simulink model "px4demo_attitude_system_multi_task"  (R2014b)
settings: Solver=FixedStepDiscrete  SolverMode=SingleTasking  StartTime=0.0  StopTime=inf  RelTol=1e-3
PostLoadFcn:
  | kFactor = 1.2;
  | 
  | KpRollAttitude = 0.630138625117681 / kFactor;
  | KiRollAttitude = 0.0552303199591522 / kFactor;
  | 
  | KpPitchAttitude = 0.630138625117681 / kFactor;
  | KiPitchAttitude = 0.0552303199591522 / kFactor;
  | 
  | KpRollRate = 1.31533836563383 / kFactor;
  | KiRollRate = 0.460338699849681 / kFactor;
  | 
  | KpPitchRate = 1.31533836563383 / kFactor;
  | KiPitchRate = 0.460338699849681 / kFactor;
  | 
  | KpYawRate = 1.31533836563383 / kFactor;
  | KiYawRate = 0.460338699849681 / kFactor;
undefined symbols (not defined in the file): PX4_TUNE_ENUM, RGBLED_COLOR_ENUM, RGBLED_MODE_ENUM
libraries: simulink x6, pixhawk_sllib x6
settings Model: SimulationMode=external  ExtModeTrigDuration=800  ExtModeArchiveFileName=EXT_mode_log  ExtModeArchiveDirName=C:\Pixhawk_Branch_Experiment\Ext_mode_bkgnd\Data_Logging  ExtModeAddSuffixToVar=on  ExtModeWriteAllDataToWs=on  ExtModeLogAll=off  Creator=Adam  LastModifiedBy=darenlee
settings SolverCC: AutoInsertRateTranBlk=on
settings OptimizationCC: InlineParams=on  OptimizeModelRefInitCode=on  LifeSpan=1  MaxStackSize=64
settings HardwareCC: ProdLargestAtomicInteger=Long  ProdLargestAtomicFloat=Double  ProdEndianess=LittleEndian  ProdHWDeviceType=ARM Compatible->ARM Cortex
settings RTWCC: SystemTargetFile=ert.tlc  TemplateMakefile=ert_default_tmf  Description=Embedded Coder  GenerateReport=on  ProcessScript=ert_make_rtw_hook  Toolchain=Pixhawk Toolchain  IncludeHyperlinkInReport=on  LaunchReport=on  GenerateTraceReport=on  GenerateTraceReportSl=on  GenerateTraceReportSf=on  GenerateTraceReportEml=on  GenerateCodeMetricsReport=on
settings CodeAppCC: IgnoreCustomStorageClasses=off
settings ERTTargetCC: CodeReplacementLibrary=GCC ARM Cortex-A9  ExtMode=on  ExtModeTransport=1  ExtModeMexFile=ext_serial_win32_comm  ExtModeMexArgs=1 8 57600 10  ERTCustomFileTemplate=PX4_codertarget_file_process.tlc

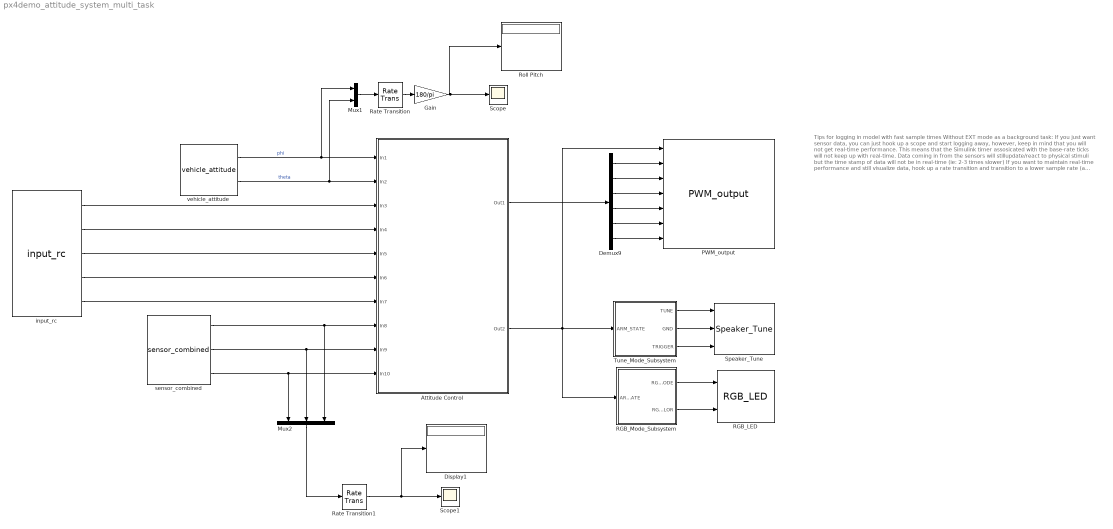
== system px4demo_attitude_system_multi_task ==
  note: Tips for logging in model with fast sample times
      |
      | Without EXT mode as a background task:
      | If you just want sensor data, you can just hook up a scope and start logging away, however, keep in mind that you will not get real-time performance. This means that the Simulink timer assosicated with the base-rate ticks will not keep up with real-time. Data coming in from the sensors will stillupdate/react to physical stimuli but the time stamp of data will not be in real-time (ie: 2-3 times slower)
      |
      | If you want to maintain real-time performance and still visualize data, hook up a rate transition and transition to a lower sample rate (a factor of 10 lower) and set the duration size to a value that will not cause the clock to slow down that much
      |
      | Recall that duration is the number of base-rate 'ticks' of data to give back. Sometimes if you set the duration too low data fails to come in for a specified sample rate. For instance, if we chose a duration value of 1:
      | 1 * 0.004 = 0.004 seconds worth of data
      | What will the lower sample (0.04s) scope show?
      | int( 0.004/0.04 ) = 0.. if we check the scope we see no data
      |
      | However, if we chose a duration value of 20
      | 400*0.004 = 1.6 seconds worth of data from base-rate
      | 1.60 / 0.04 = 40 points of data on the lower sample time scopes
      |
      | In other words, ensure the number of duration ticks gives you enough data
      | points to view on the lower sample rates, otherwise you wont see any data at all. Consult the documentation for more detail
      |
      | Using EXT mode with background task enabled
      |
      | This model has already been configured to use a background task and already uses a lot of the tips described in the above steps. With background tasking, the base-rate task is not encumbered by having to run external mode tasks at the same time, instead, EXT mode is now running in the background on another task being paced at 10 Hz. This can greatly help with real-time performance. Sometimes you may want to use the default behavior if you only have a single sample-time running at a slow rate - if you want data to come in faster or as fast as the model's sample-time then you'll want to use default behavior. On the other hand, if your model is running with multiple rates at varying speeds, you will want to pick the back-ground task option
  Attitude Control : Subsystem
  Demux9 : Demux  Outputs=6
  Display1 : Display
  Gain : Gain  Gain=180/pi
  Mux1 : Mux  Inputs=2
  Mux2 : Mux  Inputs=3
  PWM_output : pixhawk_sllib/PWM_output  show_pwm1=on  show_pwm2=on  show_pwm3=on  show_pwm4=on  show_pwm5=on  show_pwm6=on  show_pwm7=off  show_pwm8=off
  RGB_LED : pixhawk_sllib/RGB_LED
  RGB_Mode_Subsystem : Subsystem
  Rate Transition : RateTransition  OutPortSampleTime=0.04
  Rate Transition1 : RateTransition  OutPortSampleTime=0.04
  Roll Pitch : Display
  Scope : Scope
      settings: TimeRange=2  YMin=-1  YMax=1
  Scope1 : Scope
      settings: TimeRange=1.5  YMin=-1  YMax=1
  Speaker_Tune : pixhawk_sllib/Speaker_Tune
  Tune_Mode_Subsystem : Subsystem
  input_rc : pixhawk_sllib/input_rc  sampletime=1/250  channel1=on  channel2=on  channel3=on  channel4=on  channel5=on  channel6=off  channel7=off  channel8=off  ch_count=off  rssi=off  rc_failsafe=off  rc_lost=off  rc_inputsource=off
  sensor_combined : pixhawk_sllib/sensor_combined  sampletime=1/250  show_mag=off  show_acc=off  show_gyro=on  show_baro=off  show_ts=off
  vehicle_attitude : pixhawk_sllib/vehicle_attitude  sampletime=1/250  show_r=on  show_p=on  show_y=off  show_q=off
  wires:
  Demux9/6 -> PWM_output/7
  Demux9/5 -> PWM_output/6
  Demux9/4 -> PWM_output/5
  Demux9/2 -> PWM_output/3
  Demux9/3 -> PWM_output/4
  RGB_Mode_Subsystem/1(RGB_MODE) -> RGB_LED/1
  RGB_Mode_Subsystem/2(RGB_COLOR) -> RGB_LED/2
  Tune_Mode_Subsystem/1(TUNE) -> Speaker_Tune/1
  Tune_Mode_Subsystem/2(GND) -> Speaker_Tune/2
  Tune_Mode_Subsystem/3(TRIGGER) -> Speaker_Tune/3
  Attitude Control/2(Out2) -> PWM_output/1, Tune_Mode_Subsystem/1(ARM_STATE), RGB_Mode_Subsystem/1(ARM_STATE)
  vehicle_attitude/1 -> Mux1/1, Attitude Control/1(In1)  "phi"
  vehicle_attitude/2 -> Attitude Control/2(In2), Mux1/2  "theta"
  input_rc/1 -> Attitude Control/3(In3)
  input_rc/2 -> Attitude Control/4(In4)
  input_rc/3 -> Attitude Control/5(In5)
  input_rc/4 -> Attitude Control/6(In6)
  sensor_combined/1 -> Mux2/3, Attitude Control/8(In8)
  sensor_combined/2 -> Mux2/2, Attitude Control/9(In9)
  sensor_combined/3 -> Mux2/1, Attitude Control/10(In10)
  Attitude Control/1(Out1) -> Demux9/1
  Demux9/1 -> PWM_output/2
  input_rc/5 -> Attitude Control/7(In7)
  Mux1/1 -> Rate Transition/1
  Rate Transition/1 -> Gain/1
  Rate Transition1/1 -> Scope1/1, Display1/1
  Mux2/1 -> Rate Transition1/1
  Gain/1 -> Roll Pitch/1, Scope/1

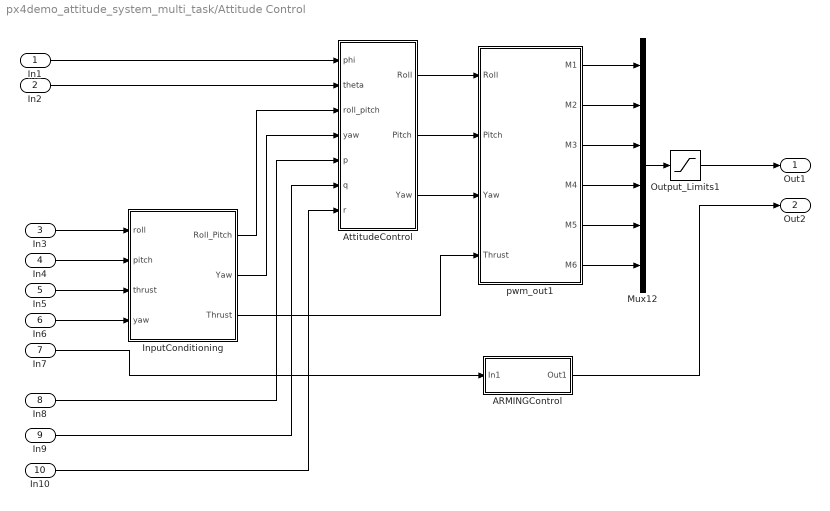
== system px4demo_attitude_system_multi_task/Attitude Control ==
  In1 : Inport
  In2 : Inport  Port=2
  In3 : Inport  Port=3
  In4 : Inport  Port=4
  In5 : Inport  Port=5
  In6 : Inport  Port=6
  In7 : Inport  Port=7
  In8 : Inport  Port=8
  In9 : Inport  Port=9
  In10 : Inport  Port=10
  ARMINGControl : Subsystem
  AttitudeControl : Subsystem
  InputConditioning : Subsystem
  Mux12 : Mux  Inputs=6
  Output_Limits1 : Saturate  UpperLimit=2000  LowerLimit=1000
  pwm_out1 : MATLAB Function  TreatAsAtomicUnit=on  SystemSampleTime=0.004
  Out1 : Outport
  Out2 : Outport  Port=2
  wires:
  ARMINGControl/1(Out1) -> Out2/1
  In6/1 -> InputConditioning/4(yaw)
  pwm_out1/4(M4) -> Mux12/4
  pwm_out1/3(M3) -> Mux12/3
  pwm_out1/2(M2) -> Mux12/2
  pwm_out1/1(M1) -> Mux12/1
  pwm_out1/5(M5) -> Mux12/5
  In7/1 -> ARMINGControl/1(In1)
  AttitudeControl/3(Yaw) -> pwm_out1/3(Yaw)
  AttitudeControl/2(Pitch) -> pwm_out1/2(Pitch)
  AttitudeControl/1(Roll) -> pwm_out1/1(Roll)
  In10/1 -> AttitudeControl/7(r)
  In9/1 -> AttitudeControl/6(q)
  In8/1 -> AttitudeControl/5(p)
  InputConditioning/2(Yaw) -> AttitudeControl/4(yaw)
  InputConditioning/1(Roll_Pitch) -> AttitudeControl/3(roll_pitch)
  In2/1 -> AttitudeControl/2(theta)
  In1/1 -> AttitudeControl/1(phi)
  InputConditioning/3(Thrust) -> pwm_out1/4(Thrust)
  Output_Limits1/1 -> Out1/1
  Mux12/1 -> Output_Limits1/1
  In4/1 -> InputConditioning/2(pitch)
  In3/1 -> InputConditioning/1(roll)
  pwm_out1/6(M6) -> Mux12/6
  In5/1 -> InputConditioning/3(thrust)

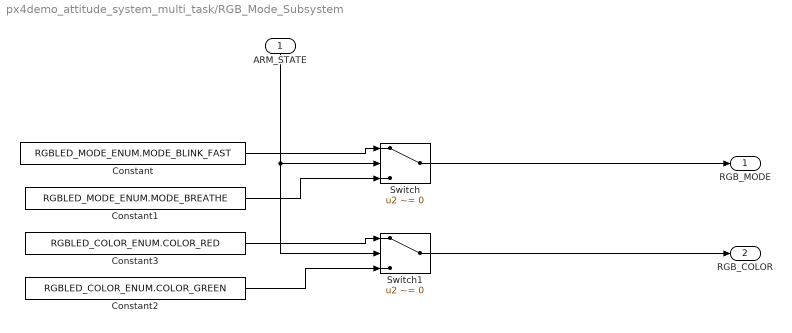
== system px4demo_attitude_system_multi_task/RGB_Mode_Subsystem ==
  ARM_STATE : Inport
  Constant : Constant  Value=RGBLED_MODE_ENUM.MODE_BLINK_FAST  OutDataTypeStr=Enum: RGBLED_MODE_ENUM
  Constant1 : Constant  Value=RGBLED_MODE_ENUM.MODE_BREATHE  OutDataTypeStr=Enum: RGBLED_MODE_ENUM
  Constant2 : Constant  Value=RGBLED_COLOR_ENUM.COLOR_GREEN  OutDataTypeStr=Enum: RGBLED_COLOR_ENUM
  Constant3 : Constant  Value=RGBLED_COLOR_ENUM.COLOR_RED  OutDataTypeStr=Enum: RGBLED_COLOR_ENUM
  Switch : Switch  Criteria=u2 ~= 0  Threshold=1500  SampleTime=1/2
  Switch1 : Switch  Criteria=u2 ~= 0  Threshold=1500  SampleTime=1/2
  RGB_MODE : Outport
  RGB_COLOR : Outport  Port=2
  wires:
  ARM_STATE/1 -> Switch1/2, Switch/2
  Constant/1 -> Switch/1
  Constant1/1 -> Switch/3
  Switch/1 -> RGB_MODE/1
  Constant3/1 -> Switch1/1
  Constant2/1 -> Switch1/3
  Switch1/1 -> RGB_COLOR/1

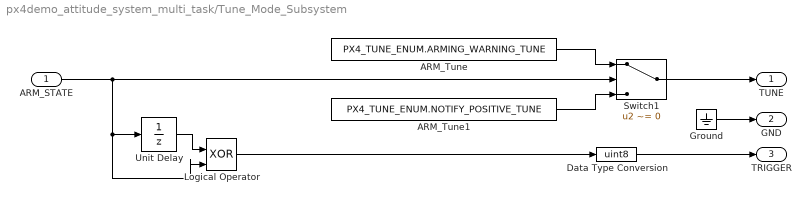
== system px4demo_attitude_system_multi_task/Tune_Mode_Subsystem ==
  ARM_STATE : Inport
  ARM_Tune : Constant  Value=PX4_TUNE_ENUM.ARMING_WARNING_TUNE  OutDataTypeStr=Enum: PX4_TUNE_ENUM
  ARM_Tune1 : Constant  Value=PX4_TUNE_ENUM.NOTIFY_POSITIVE_TUNE  OutDataTypeStr=Enum: PX4_TUNE_ENUM
  Data Type Conversion : DataTypeConversion  OutDataTypeStr=uint8
  Ground : Ground
  Logical Operator : Logic  Operator=XOR  IconShape=distinctive  AllPortsSameDT=off  OutDataTypeStr=boolean
  Switch1 : Switch  Criteria=u2 ~= 0  Threshold=1500
  Unit Delay : UnitDelay  SampleTime=-1
  TUNE : Outport
  GND : Outport  Port=2
  TRIGGER : Outport  Port=3
  wires:
  Ground/1 -> GND/1
  Data Type Conversion/1 -> TRIGGER/1
  Switch1/1 -> TUNE/1
  ARM_Tune/1 -> Switch1/1
  ARM_Tune1/1 -> Switch1/3
  ARM_STATE/1 -> Logical Operator/2, Unit Delay/1, Switch1/2
  Unit Delay/1 -> Logical Operator/1
  Logical Operator/1 -> Data Type Conversion/1

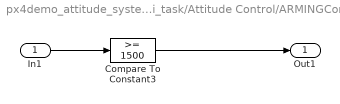
== system px4demo_attitude_system_multi_task/Attitude Control/ARMINGControl ==
  In1 : Inport
  Compare To Constant3 : simulink/Logic and Bit Operations/Compare To Constant  relop=>=  const=1500  OutDataTypeStr=boolean
  Out1 : Outport
  wires:
  Compare To Constant3/1 -> Out1/1
  In1/1 -> Compare To Constant3/1

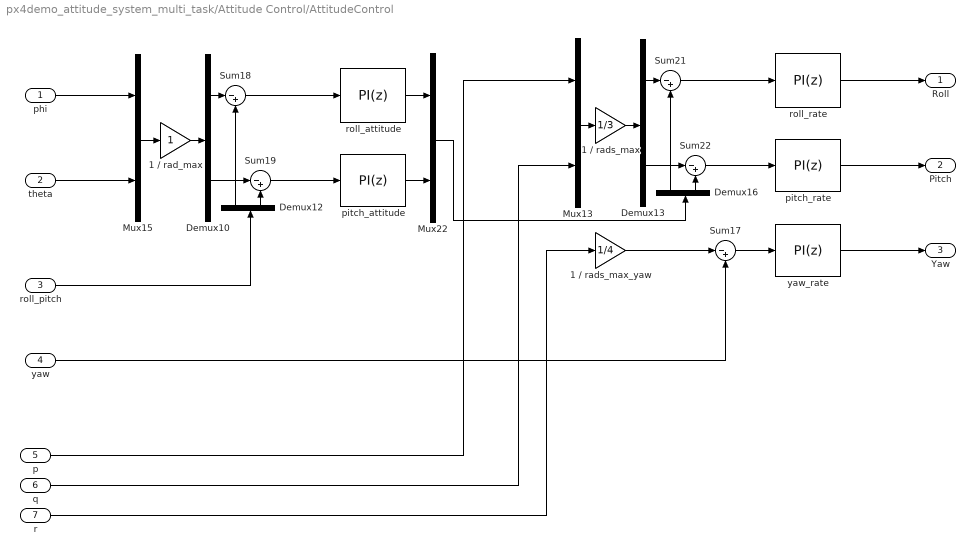
== system px4demo_attitude_system_multi_task/Attitude Control/AttitudeControl ==
  phi : Inport
  theta : Inport  Port=2
  roll_pitch : Inport  Port=3
  yaw : Inport  Port=4
  p : Inport  Port=5
  q : Inport  Port=6
  r : Inport  Port=7
  1 / rad_max : Gain
  1 / rads_max : Gain  Gain=1/3
  1 / rads_max_yaw : Gain  Gain=1/4
  Demux{10,12..13,16} (4 alike) : Demux  Outputs=2
  Mux13 : Mux  Inputs=2
  Mux15 : Mux  Inputs=2
  Mux22 : Mux  Inputs=2
  Sum{17..19,21..22} (5 alike) : Sum  Inputs=|-+
  pitch_attitude : simulink/Continuous/PID Controller  Controller=PI  TimeDomain=Discrete-time  SampleTime=-1  IntegratorMethod=Forward Euler  FilterMethod=Forward Euler  Form=Parallel  P=KpPitchAttitude  I=KiPitchAttitude  D=0.01  N=100  InitialConditionSource=internal  InitialConditionForIntegrator=0  InitialConditionForFilter=0  ExternalReset=none  LimitOutput=on  UpperSaturationLimit=1  LowerSaturationLimit=-1  LinearizeAsGain=on  AntiWindupMode=back-calculation  Kb=1  TrackingMode=off  Kt=1  PParamMin=[]  PParamMax=[]  IParamMin=[]  IParamMax=[]  DParamMin=[]  DParamMax=[]  NParamMin=[]  NParamMax=[]  KbParamMin=[]  KbParamMax=[]  KtParamMin=[]  KtParamMax=[]  POutMin=[]  POutMax=[]  IOutMin=[]  IOutMax=[]  DOutMin=[]  DOutMax=[]  NOutMin=[]  NOutMax=[]  KbOutMin=[]  KbOutMax=[]  KtOutMin=[]  KtOutMax=[]  IntegratorOutMin=[]  IntegratorOutMax=[]  FilterOutMin=[]  FilterOutMax=[]  SumOutMin=[]  SumOutMax=[]  SumI1OutMin=[]  SumI1OutMax=[]  SumI2OutMin=[]  SumI2OutMax=[]  SumI3OutMin=[]  SumI3OutMax=[]  SumDOutMin=[]  SumDOutMax=[]  SaturationOutMin=[]  SaturationOutMax=[]  IntegratorContinuousStateAttributes=''  IntegratorStateMustResolveToSignalObject=off  IntegratorRTWStateStorageClass=Auto  FilterContinuousStateAttributes=''  FilterStateMustResolveToSignalObject=off  FilterRTWStateStorageClass=Auto  DifferentiatorICPrevScaledInput=0  DifferentiatorOutMin=[]  DifferentiatorOutMax=[]  UseFilter=on
  pitch_rate : simulink/Continuous/PID Controller  Controller=PI  TimeDomain=Discrete-time  SampleTime=-1  IntegratorMethod=Forward Euler  FilterMethod=Forward Euler  Form=Parallel  P=KpPitchRate  I=KiPitchRate  D=0.0024  N=100  InitialConditionSource=internal  InitialConditionForIntegrator=0  InitialConditionForFilter=0  ExternalReset=none  LimitOutput=on  UpperSaturationLimit=1  LowerSaturationLimit=-1  LinearizeAsGain=on  AntiWindupMode=back-calculation  Kb=1  TrackingMode=off  Kt=1  PParamMin=[]  PParamMax=[]  IParamMin=[]  IParamMax=[]  DParamMin=[]  DParamMax=[]  NParamMin=[]  NParamMax=[]  KbParamMin=[]  KbParamMax=[]  KtParamMin=[]  KtParamMax=[]  POutMin=[]  POutMax=[]  IOutMin=[]  IOutMax=[]  DOutMin=[]  DOutMax=[]  NOutMin=[]  NOutMax=[]  KbOutMin=[]  KbOutMax=[]  KtOutMin=[]  KtOutMax=[]  IntegratorOutMin=[]  IntegratorOutMax=[]  FilterOutMin=[]  FilterOutMax=[]  SumOutMin=[]  SumOutMax=[]  SumI1OutMin=[]  SumI1OutMax=[]  SumI2OutMin=[]  SumI2OutMax=[]  SumI3OutMin=[]  SumI3OutMax=[]  SumDOutMin=[]  SumDOutMax=[]  SaturationOutMin=[]  SaturationOutMax=[]  IntegratorContinuousStateAttributes=''  IntegratorStateMustResolveToSignalObject=off  IntegratorRTWStateStorageClass=Auto  FilterContinuousStateAttributes=''  FilterStateMustResolveToSignalObject=off  FilterRTWStateStorageClass=Auto  DifferentiatorICPrevScaledInput=0  DifferentiatorOutMin=[]  DifferentiatorOutMax=[]  UseFilter=on
  roll_attitude : simulink/Continuous/PID Controller  Controller=PI  TimeDomain=Discrete-time  SampleTime=-1  IntegratorMethod=Forward Euler  FilterMethod=Forward Euler  Form=Parallel  P=KpRollAttitude  I=KiRollAttitude  D=0.01  N=100  InitialConditionSource=internal  InitialConditionForIntegrator=0  InitialConditionForFilter=0  ExternalReset=none  LimitOutput=on  UpperSaturationLimit=1  LowerSaturationLimit=-1  LinearizeAsGain=on  AntiWindupMode=back-calculation  Kb=1  TrackingMode=off  Kt=1  PParamMin=[]  PParamMax=[]  IParamMin=[]  IParamMax=[]  DParamMin=[]  DParamMax=[]  NParamMin=[]  NParamMax=[]  KbParamMin=[]  KbParamMax=[]  KtParamMin=[]  KtParamMax=[]  POutMin=[]  POutMax=[]  IOutMin=[]  IOutMax=[]  DOutMin=[]  DOutMax=[]  NOutMin=[]  NOutMax=[]  KbOutMin=[]  KbOutMax=[]  KtOutMin=[]  KtOutMax=[]  IntegratorOutMin=[]  IntegratorOutMax=[]  FilterOutMin=[]  FilterOutMax=[]  SumOutMin=[]  SumOutMax=[]  SumI1OutMin=[]  SumI1OutMax=[]  SumI2OutMin=[]  SumI2OutMax=[]  SumI3OutMin=[]  SumI3OutMax=[]  SumDOutMin=[]  SumDOutMax=[]  SaturationOutMin=[]  SaturationOutMax=[]  IntegratorContinuousStateAttributes=''  IntegratorStateMustResolveToSignalObject=off  IntegratorRTWStateStorageClass=Auto  FilterContinuousStateAttributes=''  FilterStateMustResolveToSignalObject=off  FilterRTWStateStorageClass=Auto  DifferentiatorICPrevScaledInput=0  DifferentiatorOutMin=[]  DifferentiatorOutMax=[]  UseFilter=on
  roll_rate : simulink/Continuous/PID Controller  Controller=PI  TimeDomain=Discrete-time  SampleTime=-1  IntegratorMethod=Forward Euler  FilterMethod=Forward Euler  Form=Parallel  P=KpRollRate  I=KiRollRate  D=0.0024  N=100  InitialConditionSource=internal  InitialConditionForIntegrator=0  InitialConditionForFilter=0  ExternalReset=none  LimitOutput=on  UpperSaturationLimit=1  LowerSaturationLimit=-1  LinearizeAsGain=on  AntiWindupMode=back-calculation  Kb=1  TrackingMode=off  Kt=1  PParamMin=[]  PParamMax=[]  IParamMin=[]  IParamMax=[]  DParamMin=[]  DParamMax=[]  NParamMin=[]  NParamMax=[]  KbParamMin=[]  KbParamMax=[]  KtParamMin=[]  KtParamMax=[]  POutMin=[]  POutMax=[]  IOutMin=[]  IOutMax=[]  DOutMin=[]  DOutMax=[]  NOutMin=[]  NOutMax=[]  KbOutMin=[]  KbOutMax=[]  KtOutMin=[]  KtOutMax=[]  IntegratorOutMin=[]  IntegratorOutMax=[]  FilterOutMin=[]  FilterOutMax=[]  SumOutMin=[]  SumOutMax=[]  SumI1OutMin=[]  SumI1OutMax=[]  SumI2OutMin=[]  SumI2OutMax=[]  SumI3OutMin=[]  SumI3OutMax=[]  SumDOutMin=[]  SumDOutMax=[]  SaturationOutMin=[]  SaturationOutMax=[]  IntegratorContinuousStateAttributes=''  IntegratorStateMustResolveToSignalObject=off  IntegratorRTWStateStorageClass=Auto  FilterContinuousStateAttributes=''  FilterStateMustResolveToSignalObject=off  FilterRTWStateStorageClass=Auto  DifferentiatorICPrevScaledInput=0  DifferentiatorOutMin=[]  DifferentiatorOutMax=[]  UseFilter=on
  yaw_rate : simulink/Continuous/PID Controller  Controller=PI  TimeDomain=Discrete-time  SampleTime=-1  IntegratorMethod=Forward Euler  FilterMethod=Forward Euler  Form=Parallel  P=KpYawRate  I=KiYawRate  D=0  N=100  InitialConditionSource=internal  InitialConditionForIntegrator=0  InitialConditionForFilter=0  ExternalReset=none  LimitOutput=on  UpperSaturationLimit=1  LowerSaturationLimit=-1  LinearizeAsGain=on  AntiWindupMode=back-calculation  Kb=1  TrackingMode=off  Kt=1  PParamMin=[]  PParamMax=[]  IParamMin=[]  IParamMax=[]  DParamMin=[]  DParamMax=[]  NParamMin=[]  NParamMax=[]  KbParamMin=[]  KbParamMax=[]  KtParamMin=[]  KtParamMax=[]  POutMin=[]  POutMax=[]  IOutMin=[]  IOutMax=[]  DOutMin=[]  DOutMax=[]  NOutMin=[]  NOutMax=[]  KbOutMin=[]  KbOutMax=[]  KtOutMin=[]  KtOutMax=[]  IntegratorOutMin=[]  IntegratorOutMax=[]  FilterOutMin=[]  FilterOutMax=[]  SumOutMin=[]  SumOutMax=[]  SumI1OutMin=[]  SumI1OutMax=[]  SumI2OutMin=[]  SumI2OutMax=[]  SumI3OutMin=[]  SumI3OutMax=[]  SumDOutMin=[]  SumDOutMax=[]  SaturationOutMin=[]  SaturationOutMax=[]  IntegratorContinuousStateAttributes=''  IntegratorStateMustResolveToSignalObject=off  IntegratorRTWStateStorageClass=Auto  FilterContinuousStateAttributes=''  FilterStateMustResolveToSignalObject=off  FilterRTWStateStorageClass=Auto  DifferentiatorICPrevScaledInput=0  DifferentiatorOutMin=[]  DifferentiatorOutMax=[]  UseFilter=on
  Roll : Outport
  Pitch : Outport  Port=2
  Yaw : Outport  Port=3
  wires:
  r/1 -> 1 / rads_max_yaw/1
  q/1 -> Mux13/2
  Mux22/1 -> Demux16/1
  yaw_rate/1 -> Yaw/1
  phi/1 -> Mux15/1
  Mux15/1 -> 1 / rad_max/1
  theta/1 -> Mux15/2
  1 / rads_max_yaw/1 -> Sum17/1
  roll_rate/1 -> Roll/1
  Sum19/1 -> pitch_attitude/1
  pitch_attitude/1 -> Mux22/2
  roll_attitude/1 -> Mux22/1
  Demux16/1 -> Sum21/2
  yaw/1 -> Sum17/2
  roll_pitch/1 -> Demux12/1
  Demux16/2 -> Sum22/2
  Demux12/1 -> Sum18/2
  Demux12/2 -> Sum19/2
  p/1 -> Mux13/1
  Demux10/1 -> Sum18/1
  Demux10/2 -> Sum19/1
  1 / rad_max/1 -> Demux10/1
  Sum18/1 -> roll_attitude/1
  pitch_rate/1 -> Pitch/1
  Mux13/1 -> 1 / rads_max/1
  Sum22/1 -> pitch_rate/1
  Sum17/1 -> yaw_rate/1
  Demux13/1 -> Sum21/1
  Demux13/2 -> Sum22/1
  1 / rads_max/1 -> Demux13/1
  Sum21/1 -> roll_rate/1

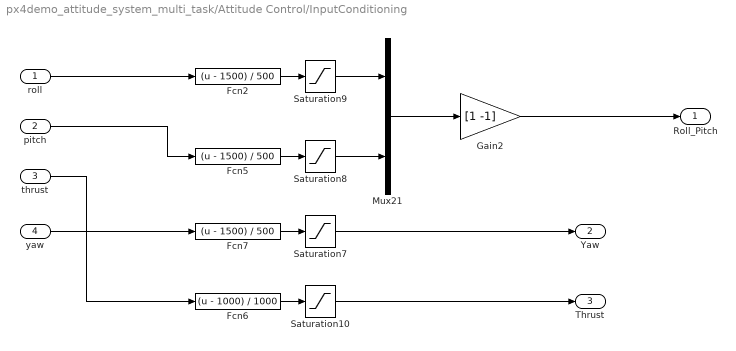
== system px4demo_attitude_system_multi_task/Attitude Control/InputConditioning ==
  roll : Inport
  pitch : Inport  Port=2
  thrust : Inport  Port=3
  yaw : Inport  Port=4
  Fcn2 : Fcn  Expr=(u - 1500) / 500
  Fcn5 : Fcn  Expr=(u - 1500) / 500
  Fcn6 : Fcn  Expr=(u - 1000) / 1000
  Fcn7 : Fcn  Expr=(u - 1500) / 500
  Gain2 : Gain  Gain=[1 -1]
  Mux21 : Mux  Inputs=2
  Saturation10 : Saturate  UpperLimit=1  LowerLimit=0
  Saturation7 : Saturate  UpperLimit=1  LowerLimit=-1
  Saturation8 : Saturate  UpperLimit=1  LowerLimit=-1
  Saturation9 : Saturate  UpperLimit=1  LowerLimit=-1
  Roll_Pitch : Outport
  Yaw : Outport  Port=2
  Thrust : Outport  Port=3
  wires:
  Saturation10/1 -> Thrust/1
  Saturation7/1 -> Yaw/1
  Gain2/1 -> Roll_Pitch/1
  Mux21/1 -> Gain2/1
  Saturation8/1 -> Mux21/2
  Fcn6/1 -> Saturation10/1
  thrust/1 -> Fcn6/1
  Fcn2/1 -> Saturation9/1
  Fcn5/1 -> Saturation8/1
  Saturation9/1 -> Mux21/1
  Fcn7/1 -> Saturation7/1
  yaw/1 -> Fcn7/1
  pitch/1 -> Fcn5/1
  roll/1 -> Fcn2/1

== matlab function px4demo_attitude_system_multi_task/Attitude Control/pwm_out1 ==
  data: Roll input; M1 output; Pitch input; Yaw input; Thrust input; M2 output; M3 output; M4 output; M5 output; M6 output
function [M1, M2, M3, M4, M5, M6] = motor_mixer(Roll, Pitch, Yaw, Thrust)

idle_PWM = 1000;

% Quad X
% M1 = ((Roll + Pitch - Yaw) / 2 * Thrust + Thrust) * 1000 + idle_PWM;
% M2 = ((-Roll + Pitch + Yaw) / 2 * Thrust + Thrust) * 1000 + idle_PWM;
% M3 = ((-Roll - Pitch - Yaw) / 2 * Thrust + Thrust) * 1000 + idle_PWM;
% M4 = ((Roll - Pitch + Yaw) / 2 * Thrust + Thrust) * 1000 + idle_PWM;
% M5 = 1000;
% M6 = 1000;
% M7 = 1000;
% M8 = 1000;

% Quad +
% M1 = ((Pitch - Yaw) * Thrust / 2 + Thrust) * 1000 + idle_PWM;
% M2 = ((-Roll + Yaw) * Thrust / 2 + Thrust) * 1000 + idle_PWM;
% M3 = ((-Pitch - Yaw) * Thrust / 2 + Thrust) * 1000 + idle_PWM;
% M4 = ((Roll + Yaw) * Thrust / 2 + Thrust) * 1000 + idle_PWM;
% M5 = 1000;
% M6 = 1000;
% M7 = 1000;
% M8 = 1000;

% Hex X
% M1 = ((Pitch + Roll / 2 - Yaw) * Thrust / 2 + Thrust) * 1000 + idle_PWM;
% M2 = ((Pitch - Roll / 2 + Yaw) * Thrust / 2 + Thrust) * 1000 + idle_PWM;
% M3 = ((-Roll - Yaw) * Thrust / 2 + Thrust) * 1000 + idle_PWM;
% M4 = ((-Pitch - Roll / 2 + Yaw) * Thrust / 2 + Thrust) * 1000 + idle_PWM;
% M5 = ((-Pitch + Roll / 2 - Yaw) * Thrust / 2 + Thrust) * 1000 + idle_PWM;
% M6 = ((Roll + Yaw) * Thrust / 2 + Thrust) * 1000 + idle_PWM;
% M7 = 1000;
% M8 = 1000;

% My Hex X (From Adam)
% 1M3 = ((-Roll - Yaw) * Thrust / 2 + Thrust) * 1000 + idle_PWM;
% 2M6 = ((Roll + Yaw) * Thrust / 2 + Thrust) * 1000 + idle_PWM;
% 3M1 = ((Pitch + Roll / 2 - Yaw) * Thrust / 2 + Thrust) * 1000 + idle_PWM;
% 4M4 = ((-Pitch - Roll / 2 + Yaw) * Thrust / 2 + Thrust) * 1000 + idle_PWM;
% 5M2 = ((Pitch - Roll / 2 + Yaw) * Thrust / 2 + Thrust) * 1000 + idle_PWM;
% 6M5 = ((-Pitch + Roll / 2 - Yaw) * Thrust / 2 + Thrust) * 1000 + idle_PWM;
M1 = ((-Roll - Yaw) * Thrust / 3 + Thrust) * 1000 + idle_PWM;
M2 = ((Roll + Yaw) * Thrust / 3 + Thrust) * 1000 + idle_PWM;
M3 = ((Pitch + Roll / 2 - Yaw) * Thrust / 3 + Thrust) * 1000 + idle_PWM;
M4 = ((-Pitch - Roll / 2 + Yaw) * Thrust / 3 + Thrust) * 1000 + idle_PWM;
M5 = ((Pitch - Roll / 2 + Yaw) * Thrust / 3 + Thrust) * 1000 + idle_PWM;
M6 = ((-Pitch + Roll / 2 - Yaw) * Thrust / 3 + Thrust) * 1000 + idle_PWM;

% My Hex X (Version 2)
% Roll/Yaw
% M1 = ((-Roll - Yaw) * Thrust / 2 + Thrust) * 1000 + idle_PWM;
% M2 = ((Roll + Yaw) * Thrust / 2 + Thrust) * 1000 + idle_PWM;
% % + Pitch/Roll
% M6 = ((Pitch + Roll / 2 - Yaw) * Thrust / 2 + Thrust) * 1000 + idle_PWM;
% M4 = ((Pitch - Roll / 2 + Yaw) * Thrust / 2 + Thrust) * 1000 + idle_PWM;
% % - Pitch/Roll
% M5 = ((-Pitch - Roll / 2 + Yaw) * Thrust / 2 + Thrust) * 1000 + idle_PWM;
% M3 = ((-Pitch + Roll / 2 - Yaw) * Thrust / 2 + Thrust) * 1000 + idle_PWM;

% My Hex (Version 3)
